simulink model "Luenberger"  (R2016a)
settings: Solver=FixedStepAuto  StartTime=0.0  StopTime=2  FixedStep=ts/20  RelTol=1e-3
values from neighbouring files (symbols this model uses):
  B = [B11 0; 0 B22; 0 0; 0 0]    [Luenberger_Parameters.m]
  B_m = [B11_m 0; 0 B22_m; 0 0; 0 0]    [Luenberger_Parameters.m]
  F = 0    [Luenberger_Parameters.m]
  J = 0.047    [Luenberger_Parameters.m]
  Lm = 0.1290    (= 0.129)    [Luenberger_Parameters.m]
  Lm_m = -err_per*Lm+Lm    (= 0.12642)    [Luenberger_Parameters.m]
  Lr = 0.1370    (= 0.137)    [Luenberger_Parameters.m]
  Lr_m = -err_per*Lr+Lr    (= 0.13426)    [Luenberger_Parameters.m]
  Ls = 0.1370    (= 0.137)    [Luenberger_Parameters.m]
  Ls_m = -err_per*Ls+Ls    (= 0.13426)    [Luenberger_Parameters.m]
  n_sync = 1500    [Luenberger_Parameters.m]
  p = 2    [Luenberger_Parameters.m]
  Rr = 1.8300    (= 1.83)    [Luenberger_Parameters.m]
  Rr_m = err_per*Rr+Rr    (= 1.8666)    [Luenberger_Parameters.m]
  Rs = 2.1900    (= 2.19)    [Luenberger_Parameters.m]
  Rs_m = err_per*Rs+Rs    (= 2.2338)    [Luenberger_Parameters.m]
  T_lim = 19    [Luenberger_Parameters.m]
  Tr_m = Lr_m/Rr_m    (= 0.0719275688417)    [Luenberger_Parameters.m]
  ts = 1/fs    (= 6.66666666667e-05)    [Luenberger_Parameters.m]
  Udc = 310    [Luenberger_Parameters.m]
undefined symbols (not defined in the file or in its folder): n_rated
settings Model: SimulationMode=accelerator  Creator=Administrator  LastModifiedBy=DELL
settings DataIOCC: LimitDataPoints=on  SaveFormat=Array  SignalLoggingSaveFormat=ModelDataLogs
settings OptimizationCC: ExpressionDepthLimit=2147483647
settings DebuggingCC: UnderspecifiedInitializationDetection=Classic  MergeDetectMultiDrivingBlocksExec=none  SolverPrmCheckMsg=warning  FcnCallInpInsideContextMsg=UseLocalSettings  StateNameClashWarn=warning
settings HardwareCC: ProdBitPerPointer=32  ProdLargestAtomicFloat=None  ProdIntDivRoundTo=Undefined  ProdEndianess=Unspecified  ProdWordSize=32  ProdHWDeviceType=32-bit Generic
settings ModelReferenceCC: PropagateSignalLabelsOutOfModel=off
settings GRTTargetCC: CombineOutputUpdateFcns=off  GRTInterface=on
settings ConfigComp: CovModelRefEnable=Off  CovSFcnEnable=off

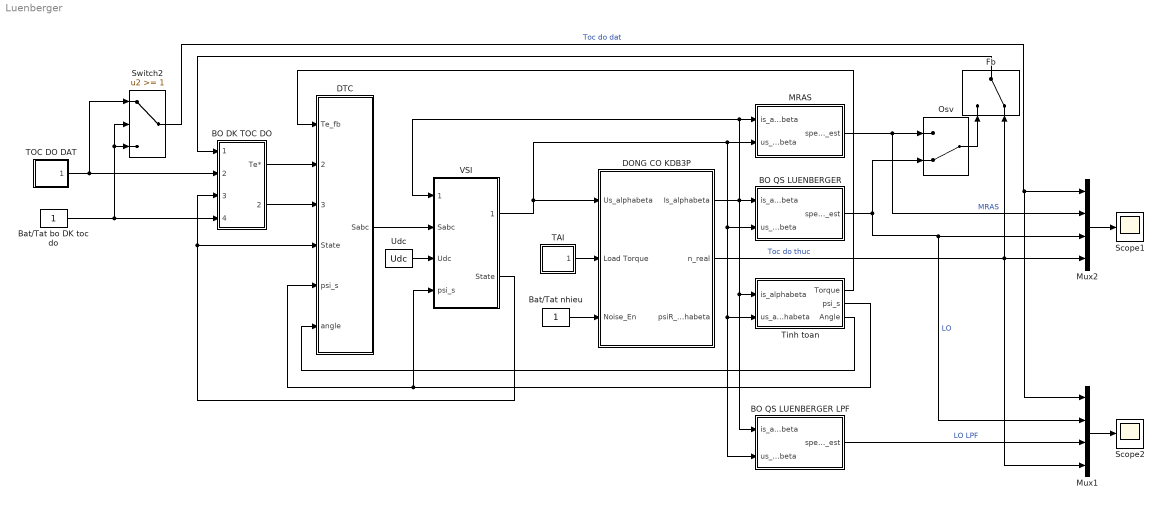
== system Luenberger ==
  BO DK TOC DO : Subsystem
  BO QS LUENBERGER : Subsystem
  BO QS LUENBERGER LPF : Subsystem
  Bat/Tat bo DK toc do : Constant
  Bat/Tat nhieu : Constant
  DONG CO KDB3P : Subsystem
  DTC : Subsystem
  Fb : ManualSwitch  CurrentSetting=0
  MRAS : Subsystem
  Mux1 : Mux
  Mux2 : Mux
  Osv : ManualSwitch  CurrentSetting=0
  Scope1 : Scope
  Scope2 : Scope
  Switch2 : Switch  Threshold=1
  TAI : Subsystem
  TOC DO DAT : Subsystem
  Tinh toan : Subsystem
  Udc : Constant  Value=Udc
  VSI : Subsystem
  wires:
  BO DK TOC DO/1(Te*) -> DTC/2(Te_ref)
  BO DK TOC DO/2(Flux*) -> DTC/3(Flux_ref)
  Tinh toan/1(Torque) -> DTC/1(Te_fb)
  Tinh toan/2(psi_s) -> DTC/5(psi_s), VSI/4(psi_s)
  VSI/2(State) -> DTC/4(State), BO DK TOC DO/3(State)
  Mux2/1 -> Scope1/1
  DTC/1(Sabc) -> VSI/2(Sabc)
  Udc/1 -> VSI/3(Udc)
  VSI/1(Us_alphabeta) -> MRAS/2(us_alphabeta), Tinh toan/2(us_alphabeta), BO QS LUENBERGER LPF/2(us_alphabeta), BO QS LUENBERGER/2(us_alphabeta), DONG CO KDB3P/1(Us_alphabeta)
  DONG CO KDB3P/1(Is_alphabeta) -> MRAS/1(is_alphabeta), VSI/1(is_alphabeta), BO QS LUENBERGER/1(is_alphabeta), BO QS LUENBERGER LPF/1(is_alphabeta), Tinh toan/1(is_alphabeta)
  Tinh toan/3(Angle) -> DTC/6(angle)
  Bat/Tat nhieu/1 -> DONG CO KDB3P/3(Noise_En)
  Fb/1 -> BO DK TOC DO/1(rpm_fb)
  Bat/Tat bo DK toc do/1 -> Switch2/3, Switch2/2, BO DK TOC DO/4(Enable)
  TOC DO DAT/1(Speed) -> Switch2/1, BO DK TOC DO/2(rpm_ref)
  TAI/1(Load) -> DONG CO KDB3P/2(Load Torque)
  MRAS/1(speed_est) -> Mux2/2, Osv/1  "MRAS"
  Osv/1 -> Fb/1
  Switch2/1 -> Mux1/1, Mux2/1  "Toc do dat"
  Mux1/1 -> Scope2/1
  DONG CO KDB3P/2(n_real) -> Mux1/4, Fb/2, Mux2/4  "Toc do thuc"
  BO QS LUENBERGER LPF/1(speed_est) -> Mux1/3  "LO LPF"
  BO QS LUENBERGER/1(speed_est) -> Mux1/2, Mux2/3, Osv/2  "LO"

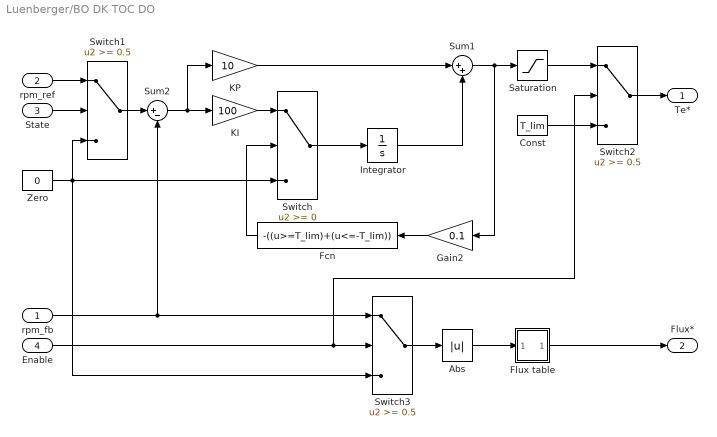
== system Luenberger/BO DK TOC DO ==
  rpm_fb : Inport
  rpm_ref : Inport  Port=2
  State : Inport  Port=3
  Enable : Inport  Port=4
  Abs : Abs  SaturateOnIntegerOverflow=on
  Const : Constant  Value=T_lim
  Fcn : Fcn  Expr=-((u>=T_lim)+(u<=-T_lim))
  Flux table : Subsystem
      mask Display: plot([0;1800;2000;2500;3000;3500], [1;1;0.90*1;0.72*1;0.6*1;0.51*1])
  Gain2 : Gain  Gain=0.1
  Integrator : Integrator  UpperSaturationLimit=T_lim  LowerSaturationLimit=-T_lim
  KI : Gain  Gain=100
  KP : Gain  Gain=10
  Saturation : Saturate  UpperLimit=T_lim  LowerLimit=-T_lim
  Sum1 : Sum  Inputs=|++
  Sum2 : Sum  Inputs=|+-
  Switch : Switch
  Switch1 : Switch  Threshold=0.5
  Switch2 : Switch  Threshold=0.5
  Switch3 : Switch  Threshold=0.5
  Zero : Constant  Value=0
  Te* : Outport
  Flux* : Outport  Port=2
  wires:
  Abs/1 -> Flux table/1(|N|)
  State/1 -> Switch1/2
  rpm_ref/1 -> Switch1/1
  Zero/1 -> Switch3/3, Switch/3, Switch1/3
  rpm_fb/1 -> Switch3/1, Sum2/2
  Switch1/1 -> Sum2/1
  Sum1/1 -> Gain2/1, Saturation/1
  KP/1 -> Sum1/1
  Fcn/1 -> Switch/2
  Gain2/1 -> Fcn/1
  Sum2/1 -> KI/1, KP/1
  Switch/1 -> Integrator/1
  KI/1 -> Switch/1
  Integrator/1 -> Sum1/2
  Saturation/1 -> Switch2/1
  Switch2/1 -> Te*/1
  Const/1 -> Switch2/3
  Flux table/1(Flux) -> Flux*/1
  Switch3/1 -> Abs/1
  Enable/1 -> Switch2/2, Switch3/2

== system Luenberger/BO QS LUENBERGER ==
  is_alphabeta : Inport
  us_alphabeta : Inport  Port=2
  Demux1 : Demux  Outputs=2
  Divide : Product  Inputs=*/
  Luenberger Adaptation Algorithm : Subsystem
  Luenberger Algorithm : Subsystem
  pole pair : Constant  Value=p
  w-->n3 : Gain  Gain=30/pi
  speed_est : Outport
  wires:
  us_alphabeta/1 -> Luenberger Algorithm/2(Us_alphabeta)
  Luenberger Adaptation Algorithm/1(wr^) -> Luenberger Algorithm/1(w_est), Divide/1
  w-->n3/1 -> speed_est/1
  Divide/1 -> w-->n3/1
  pole pair/1 -> Divide/2
  Luenberger Algorithm/1(Is_alphabeta^) -> Luenberger Adaptation Algorithm/1(is_alphabeta^)
  Luenberger Algorithm/2(PsiR_alphabeta^) -> Luenberger Adaptation Algorithm/2(psir_alphabeta^)
  is_alphabeta/1 -> Demux1/1
  Demux1/1 -> Luenberger Adaptation Algorithm/3(is_alpha), Luenberger Algorithm/3(is_alpha)
  Demux1/2 -> Luenberger Algorithm/4(is_beta), Luenberger Adaptation Algorithm/4(is_beta)

== system Luenberger/BO QS LUENBERGER LPF ==
  is_alphabeta : Inport
  us_alphabeta : Inport  Port=2
  Demux1 : Demux  Outputs=2
  Divide : Product  Inputs=*/
  Luenberger Adaptation Algorithm : Subsystem
  Luenberger Algorithm : Subsystem
  pole pair : Constant  Value=p
  w-->n3 : Gain  Gain=30/pi
  speed_est : Outport
  wires:
  us_alphabeta/1 -> Luenberger Algorithm/2(Us_alphabeta)
  Luenberger Adaptation Algorithm/1(wr^) -> Luenberger Algorithm/1(w_est), Divide/1
  w-->n3/1 -> speed_est/1
  Divide/1 -> w-->n3/1
  pole pair/1 -> Divide/2
  Luenberger Algorithm/1(Is_alphabeta^) -> Luenberger Adaptation Algorithm/1(is_alphabeta^)
  Luenberger Algorithm/2(PsiR_alphabeta^) -> Luenberger Adaptation Algorithm/2(psir_alphabeta^)
  is_alphabeta/1 -> Demux1/1
  Demux1/1 -> Luenberger Adaptation Algorithm/3(is_alpha), Luenberger Algorithm/3(is_alpha)
  Demux1/2 -> Luenberger Algorithm/4(is_beta), Luenberger Adaptation Algorithm/4(is_beta)

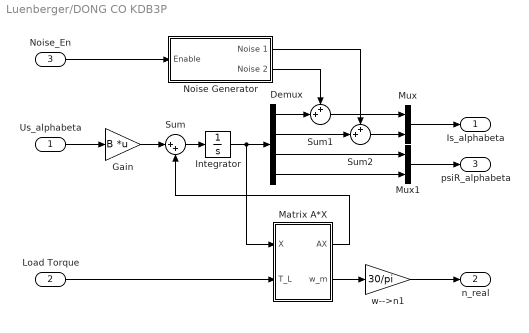
== system Luenberger/DONG CO KDB3P ==
  Us_alphabeta : Inport
  Load Torque : Inport  Port=2
  Noise_En : Inport  Port=3
  Demux : Demux
  Gain : Gain  Gain=B  Multiplication=Matrix(K*u)
  Integrator : Integrator
  Matrix A*X : Subsystem
  Mux : Mux  Inputs=2
  Mux1 : Mux  Inputs=2
  Noise Generator : Subsystem
  Sum : Sum  Inputs=|++
  Sum1 : Sum  Inputs=++|
  Sum2 : Sum  Inputs=++|
  w-->n1 : Gain  Gain=30/pi
  Is_alphabeta : Outport
  n_real : Outport  Port=2
  psiR_alphabeta : Outport  Port=3
  wires:
  Demux/3 -> Mux1/1
  Demux/4 -> Mux1/2
  Integrator/1 -> Matrix A*X/1(X), Demux/1
  Matrix A*X/1(AX) -> Sum/2
  Sum/1 -> Integrator/1
  Matrix A*X/2(w_m) -> w-->n1/1
  Us_alphabeta/1 -> Gain/1
  Gain/1 -> Sum/1
  w-->n1/1 -> n_real/1
  Load Torque/1 -> Matrix A*X/2(T_L)
  Mux1/1 -> psiR_alphabeta/1
  Mux/1 -> Is_alphabeta/1
  Demux/1 -> Sum1/2
  Demux/2 -> Sum2/2
  Sum2/1 -> Mux/2
  Sum1/1 -> Mux/1
  Noise Generator/2(Noise 2) -> Sum1/1
  Noise Generator/1(Noise 1) -> Sum2/1
  Noise_En/1 -> Noise Generator/1(Enable)

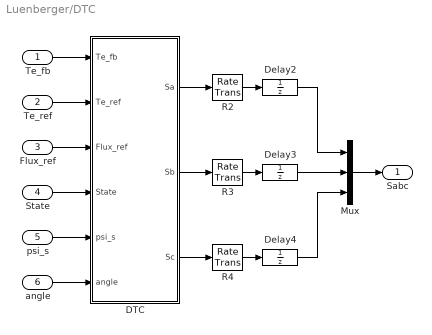
== system Luenberger/DTC ==
  Te_fb : Inport
  Te_ref : Inport  Port=2
  Flux_ref : Inport  Port=3
  State : Inport  Port=4
  psi_s : Inport  Port=5
  angle : Inport  Port=6
  DTC : MATLAB Function  TreatAsAtomicUnit=on
  Delay2 : UnitDelay  SampleTime=ts
  Delay3 : UnitDelay  SampleTime=ts
  Delay4 : UnitDelay  SampleTime=ts
  Mux : Mux  Inputs=3
  R2 : RateTransition
  R3 : RateTransition
  R4 : RateTransition
  Sabc : Outport
  wires:
  Mux/1 -> Sabc/1
  Te_fb/1 -> DTC/1(Te_fb)
  Te_ref/1 -> DTC/2(Te_ref)
  Flux_ref/1 -> DTC/3(Flux_ref)
  State/1 -> DTC/4(State)
  psi_s/1 -> DTC/5(psi_s)
  angle/1 -> DTC/6(angle)
  DTC/1(Sa) -> R2/1
  DTC/2(Sb) -> R3/1
  DTC/3(Sc) -> R4/1
  R2/1 -> Delay2/1
  R3/1 -> Delay3/1
  R4/1 -> Delay4/1
  Delay2/1 -> Mux/1
  Delay3/1 -> Mux/2
  Delay4/1 -> Mux/3

== system Luenberger/MRAS ==
  is_alphabeta : Inport
  us_alphabeta : Inport  Port=2
  CB Adaptation Algorithm : Subsystem
  CB Adaptive Model : Subsystem
  CB Estimator : Subsystem
  Divide : Product  Inputs=*/
  Lm measured : Constant  Value=Lm_m
  Lr measured : Constant  Value=Lr_m
  Ls measured : Constant  Value=Ls_m
  Rr measured : Constant  Value=Rr_m
  Rs measured : Constant  Value=Rs_m
  pole pair : Constant  Value=p
  w-->n3 : Gain  Gain=30/pi
  speed_est : Outport
  wires:
  us_alphabeta/1 -> CB Estimator/1(us_alphabeta)
  CB Adaptation Algorithm/1(w_r_CB^) -> Divide/1, CB Estimator/2(w_r_CB^), CB Adaptive Model/2(w_r_CB^)
  CB Estimator/1(is_alphabeta^) -> CB Adaptation Algorithm/1(is_alphabeta^)
  CB Adaptive Model/1(psir_alpha^) -> CB Adaptation Algorithm/3(psir_alpha^), CB Estimator/8(psir_alpha^)
  is_alphabeta/1 -> CB Adaptive Model/1(is_alphabeta), CB Adaptation Algorithm/2(is_alphabeta)
  Lm measured/1 -> CB Estimator/3("Lm_m ")
  Lr measured/1 -> CB Estimator/4(Lr_m)
  Ls measured/1 -> CB Estimator/5(Ls_m)
  Rr measured/1 -> CB Estimator/6(Rr_m)
  Rs measured/1 -> CB Estimator/7(Rs_m)
  CB Adaptive Model/2(psir_beta^) -> CB Adaptation Algorithm/4(psir_beta^), CB Estimator/9(psir_beta^)
  w-->n3/1 -> speed_est/1
  Divide/1 -> w-->n3/1
  pole pair/1 -> Divide/2

== system Luenberger/TAI ==
  note: Select=0: No load
      | Select=1: 10% load
      | Select=2: 0% -100% load
      | Select>2: 0%, 10%, 50%, 80% load
  Clock : Clock
  Load Generator : MATLAB Function  TreatAsAtomicUnit=on
  Select : Constant  Value=2
  Tmax : Constant  Value=T_lim
  Load : Outport
  wires:
  Load Generator/1(T_Load) -> Load/1
  Select/1 -> Load Generator/1(Select)
  Tmax/1 -> Load Generator/2(Tmax)
  Clock/1 -> Load Generator/3(t)

== system Luenberger/TOC DO DAT ==
  note: Select=1: 100rpm
      | Select=2: 500rpm
      | Select>2: 1000, 500, 100rpm
  Clock : Clock
  Select : Constant  Value=3
  Speed Selection : MATLAB Function  TreatAsAtomicUnit=on
  Speed : Outport
  wires:
  Speed Selection/1(Speed) -> Speed/1
  Select/1 -> Speed Selection/1(Select)
  Clock/1 -> Speed Selection/2(t)

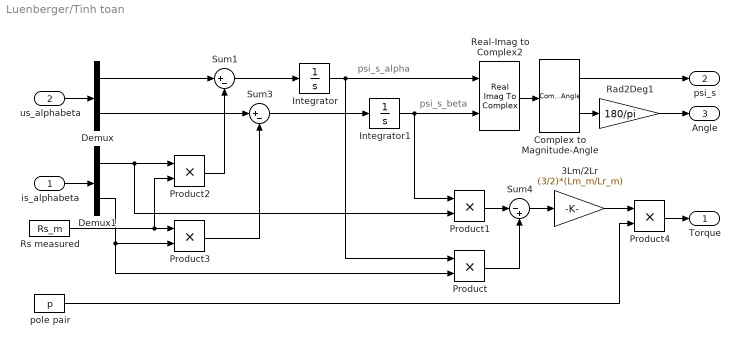
== system Luenberger/Tinh toan ==
  note: psi_s_beta
  note: psi_s_alpha
  is_alphabeta : Inport
  us_alphabeta : Inport  Port=2
  3Lm/2Lr : Gain  Gain=(3/2)*(Lm_m/Lr_m)
  Complex to Magnitude-Angle : ComplexToMagnitudeAngle
  Demux : Demux  Outputs=2
  Demux1 : Demux  Outputs=2
  Integrator : Integrator
  Integrator1 : Integrator  LimitOutput=on  UpperSaturationLimit=pi  LowerSaturationLimit=-pi
  Product{,1..4} (5 alike) : Product  RndMeth=Zero
  Rad2Deg1 : Gain  Gain=180/pi
  Real-Imag to Complex2 : RealImagToComplex
  Rs measured : Constant  Value=Rs_m
  Sum1 : Sum  Inputs=|+-
  Sum3 : Sum  Inputs=|+-
  Sum4 : Sum  Inputs=|-+
  pole pair : Constant  Value=p
  Torque : Outport
  psi_s : Outport  Port=2
  Angle : Outport  Port=3
  wires:
  Product2/1 -> Sum1/2
  Sum1/1 -> Integrator/1
  Integrator/1 -> Real-Imag to Complex2/1, Product/1
  Product3/1 -> Sum3/2
  Sum3/1 -> Integrator1/1
  Demux/2 -> Sum3/1
  Demux1/2 -> Product/2, Product3/2
  Product1/1 -> Sum4/1
  Product/1 -> Sum4/2
  Sum4/1 -> 3Lm/2Lr/1
  Real-Imag to Complex2/1 -> Complex to Magnitude-Angle/1
  Complex to Magnitude-Angle/1 -> psi_s/1
  Rs measured/1 -> Product2/2, Product3/1
  Demux/1 -> Sum1/1
  us_alphabeta/1 -> Demux/1
  is_alphabeta/1 -> Demux1/1
  Demux1/1 -> Product1/2, Product2/1
  Integrator1/1 -> Product1/1, Real-Imag to Complex2/2
  pole pair/1 -> Product4/2
  3Lm/2Lr/1 -> Product4/1
  Product4/1 -> Torque/1
  Rad2Deg1/1 -> Angle/1
  Complex to Magnitude-Angle/2 -> Rad2Deg1/1

== system Luenberger/VSI ==
  is_alphabeta : Inport
  Sabc : Inport  Port=2
  Udc : Inport  Port=3
  psi_s : Inport  Port=4
  Delay : UnitDelay  SampleTime=ts
  Demux : Demux  Outputs=3
  Demux1 : Demux  Outputs=2
  Mux : Mux  Inputs=2
  R5 : RateTransition
  VSI : MATLAB Function  TreatAsAtomicUnit=on
  Us_alphabeta : Outport
  State : Outport  Port=2
  wires:
  Udc/1 -> VSI/4(Udc)
  VSI/3(State) -> State/1, R5/1
  Delay/1 -> VSI/8(Start)
  R5/1 -> Delay/1
  Sabc/1 -> Demux/1
  Demux/1 -> VSI/1(Sa)
  Demux/2 -> VSI/2(Sb)
  psi_s/1 -> VSI/5(psi_s)
  Mux/1 -> Us_alphabeta/1
  VSI/1(u_alpha) -> Mux/1
  VSI/2(u_beta) -> Mux/2
  Demux/3 -> VSI/3(Sc)
  is_alphabeta/1 -> Demux1/1
  Demux1/1 -> VSI/6(is_alpha)
  Demux1/2 -> VSI/7(is_beta)

== system Luenberger/BO DK TOC DO/Flux table ==
  |N| : Inport
  Abs1 : Abs  SaturateOnIntegerOverflow=on
  F : Fcn  Expr=n_sync*0.78/u(1)
  Saturation : Saturate  UpperLimit=inf  LowerLimit=1500
  Flux : Outport
  wires:
  Abs1/1 -> Saturation/1
  F/1 -> Flux/1
  |N|/1 -> Abs1/1
  Saturation/1 -> F/1

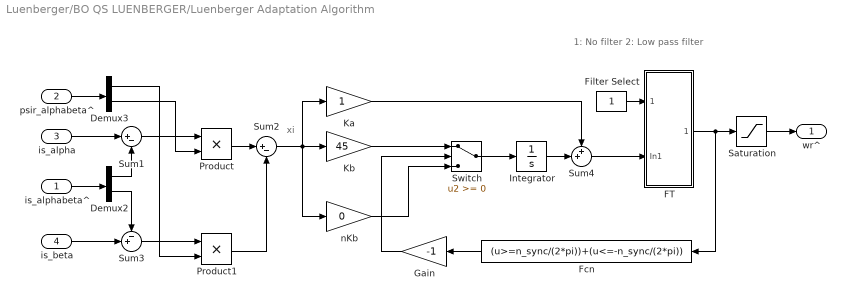
== system Luenberger/BO QS LUENBERGER/Luenberger Adaptation Algorithm ==
  note: 1: No filter
      | 2: Low pass filter
  note: xi
  is_alphabeta^ : Inport
  psir_alphabeta^ : Inport  Port=2
  is_alpha : Inport  Port=3
  is_beta : Inport  Port=4
  Demux2 : Demux  Outputs=2
  Demux3 : Demux  Outputs=2
  FT : Subsystem
  Fcn : Fcn  Expr=(u>=n_sync/(2*pi))+(u<=-n_sync/(2*pi))
  Filter Select : Constant
  Gain : Gain  Gain=-1
  Integrator : Integrator  UpperSaturationLimit=n_rated/(2*pi)  LowerSaturationLimit=-n_rated/(2*pi)
  Ka : Gain
  Kb : Gain  Gain=45
  Product : Product  RndMeth=Zero
  Product1 : Product  RndMeth=Zero
  Saturation : Saturate  UpperLimit=n_sync/(2*pi)  LowerLimit=-n_sync/(2*pi)
  Sum1 : Sum  Inputs=|+-
  Sum2 : Sum  Inputs=|+-
  Sum3 : Sum  Inputs=-+|
  Sum4 : Sum  Inputs=++|
  Switch : Switch
  nKb : Gain  Gain=0
  wr^ : Outport
  wires:
  Product1/1 -> Sum2/2
  Demux3/2 -> Product/2
  Demux3/1 -> Product1/2
  Product/1 -> Sum2/1
  Integrator/1 -> Sum4/2
  Switch/1 -> Integrator/1
  is_alphabeta^/1 -> Demux2/1
  psir_alphabeta^/1 -> Demux3/1
  Sum1/1 -> Product/1
  Sum3/1 -> Product1/1
  Filter Select/1 -> FT/1(Select)
  Demux2/2 -> Sum3/1
  is_beta/1 -> Sum3/2
  Demux2/1 -> Sum1/2
  is_alpha/1 -> Sum1/1
  Sum2/1 -> Ka/1, nKb/1, Kb/1
  Kb/1 -> Switch/1
  Fcn/1 -> Gain/1
  Gain/1 -> Switch/2
  nKb/1 -> Switch/3
  Saturation/1 -> wr^/1
  Ka/1 -> Sum4/1
  Sum4/1 -> FT/2(In1)
  FT/1(Out1) -> Fcn/1, Saturation/1

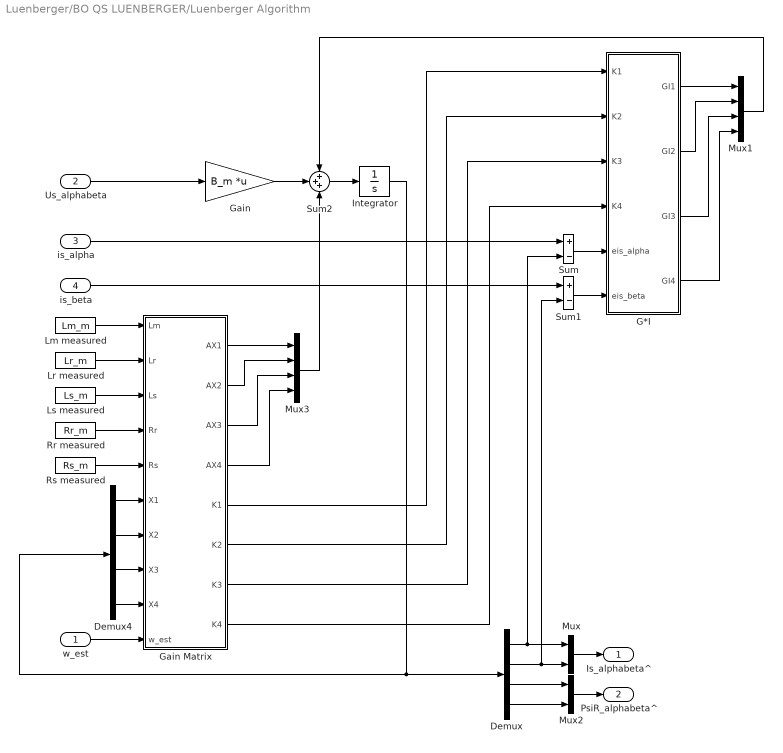
== system Luenberger/BO QS LUENBERGER/Luenberger Algorithm ==
  w_est : Inport
  Us_alphabeta : Inport  Port=2
  is_alpha : Inport  Port=3
  is_beta : Inport  Port=4
  Demux : Demux
  Demux4 : Demux
  G*I : MATLAB Function  TreatAsAtomicUnit=on
  Gain : Gain  Gain=B_m  Multiplication=Matrix(K*u)
  Gain Matrix : MATLAB Function  TreatAsAtomicUnit=on
  Integrator : Integrator
  Lm measured : Constant  Value=Lm_m
  Lr measured : Constant  Value=Lr_m
  Ls measured : Constant  Value=Ls_m
  Mux : Mux  Inputs=2
  Mux1 : Mux
  Mux2 : Mux  Inputs=2
  Mux3 : Mux
  Rr measured : Constant  Value=Rr_m
  Rs measured : Constant  Value=Rs_m
  Sum : Sum  Inputs=+-
  Sum1 : Sum  Inputs=+-
  Sum2 : Sum  Inputs=+++
  Is_alphabeta^ : Outport
  PsiR_alphabeta^ : Outport  Port=2
  wires:
  Demux/1 -> Mux/1, Sum/2
  Demux/2 -> Mux/2, Sum1/2
  Sum2/1 -> Integrator/1
  Mux1/1 -> Sum2/1
  Sum/1 -> G*I/5(eis_alpha)
  Sum1/1 -> G*I/6(eis_beta)
  G*I/1(GI1) -> Mux1/1
  G*I/2(GI2) -> Mux1/2
  G*I/3(GI3) -> Mux1/3
  G*I/4(GI4) -> Mux1/4
  is_alpha/1 -> Sum/1
  is_beta/1 -> Sum1/1
  Mux/1 -> Is_alphabeta^/1
  Demux/3 -> Mux2/1
  Demux/4 -> Mux2/2
  Mux2/1 -> PsiR_alphabeta^/1
  Gain/1 -> Sum2/2
  Us_alphabeta/1 -> Gain/1
  Integrator/1 -> Demux4/1, Demux/1
  Demux4/2 -> Gain Matrix/7(X2)
  Demux4/3 -> Gain Matrix/8(X3)
  Demux4/1 -> Gain Matrix/6(X1)
  Demux4/4 -> Gain Matrix/9(X4)
  Gain Matrix/1(AX1) -> Mux3/1
  Gain Matrix/2(AX2) -> Mux3/2
  Gain Matrix/3(AX3) -> Mux3/3
  Gain Matrix/4(AX4) -> Mux3/4
  Gain Matrix/8(K4) -> G*I/4(K4)
  Gain Matrix/7(K3) -> G*I/3(K3)
  Gain Matrix/6(K2) -> G*I/2(K2)
  Gain Matrix/5(K1) -> G*I/1(K1)
  Mux3/1 -> Sum2/3
  Lm measured/1 -> Gain Matrix/1(Lm)
  Lr measured/1 -> Gain Matrix/2(Lr)
  Ls measured/1 -> Gain Matrix/3(Ls)
  Rr measured/1 -> Gain Matrix/4(Rr)
  Rs measured/1 -> Gain Matrix/5(Rs)
  w_est/1 -> Gain Matrix/10(w_est)

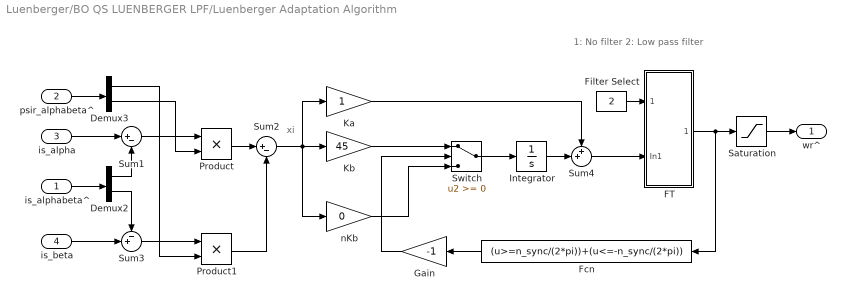
== system Luenberger/BO QS LUENBERGER LPF/Luenberger Adaptation Algorithm ==
  note: 1: No filter
      | 2: Low pass filter
  note: xi
  is_alphabeta^ : Inport
  psir_alphabeta^ : Inport  Port=2
  is_alpha : Inport  Port=3
  is_beta : Inport  Port=4
  Demux2 : Demux  Outputs=2
  Demux3 : Demux  Outputs=2
  FT : Subsystem
  Fcn : Fcn  Expr=(u>=n_sync/(2*pi))+(u<=-n_sync/(2*pi))
  Filter Select : Constant  Value=2
  Gain : Gain  Gain=-1
  Integrator : Integrator  UpperSaturationLimit=n_rated/(2*pi)  LowerSaturationLimit=-n_rated/(2*pi)
  Ka : Gain
  Kb : Gain  Gain=45
  Product : Product  RndMeth=Zero
  Product1 : Product  RndMeth=Zero
  Saturation : Saturate  UpperLimit=n_sync/(2*pi)  LowerLimit=-n_sync/(2*pi)
  Sum1 : Sum  Inputs=|+-
  Sum2 : Sum  Inputs=|+-
  Sum3 : Sum  Inputs=-+|
  Sum4 : Sum  Inputs=++|
  Switch : Switch
  nKb : Gain  Gain=0
  wr^ : Outport
  wires:
  Product1/1 -> Sum2/2
  Demux3/2 -> Product/2
  Demux3/1 -> Product1/2
  Product/1 -> Sum2/1
  Integrator/1 -> Sum4/2
  Switch/1 -> Integrator/1
  is_alphabeta^/1 -> Demux2/1
  psir_alphabeta^/1 -> Demux3/1
  Sum1/1 -> Product/1
  Sum3/1 -> Product1/1
  Filter Select/1 -> FT/1(Select)
  Demux2/2 -> Sum3/1
  is_beta/1 -> Sum3/2
  Demux2/1 -> Sum1/2
  is_alpha/1 -> Sum1/1
  Sum2/1 -> Ka/1, nKb/1, Kb/1
  Kb/1 -> Switch/1
  Fcn/1 -> Gain/1
  Gain/1 -> Switch/2
  nKb/1 -> Switch/3
  Saturation/1 -> wr^/1
  Ka/1 -> Sum4/1
  Sum4/1 -> FT/2(In1)
  FT/1(Out1) -> Fcn/1, Saturation/1

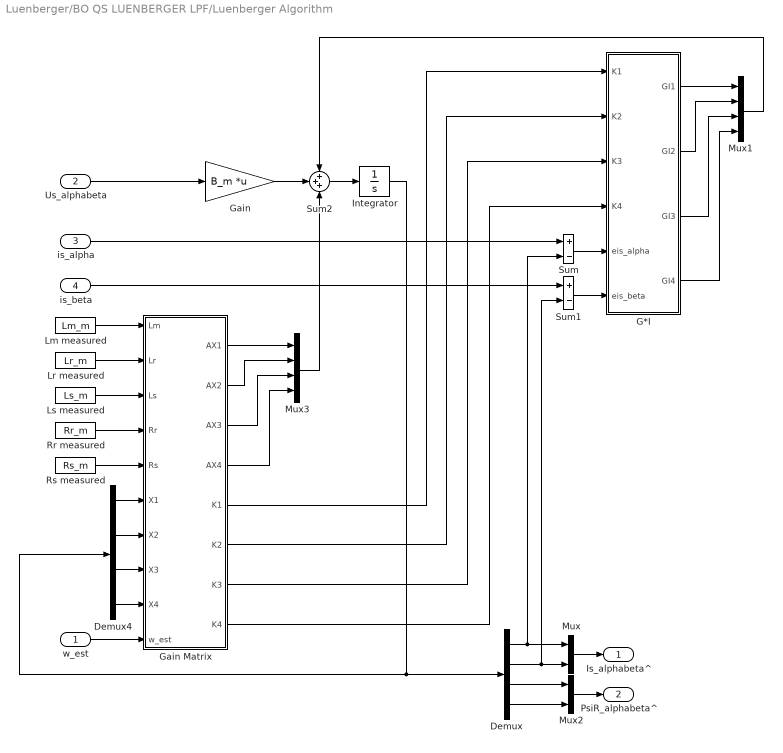
== system Luenberger/BO QS LUENBERGER LPF/Luenberger Algorithm ==
  w_est : Inport
  Us_alphabeta : Inport  Port=2
  is_alpha : Inport  Port=3
  is_beta : Inport  Port=4
  Demux : Demux
  Demux4 : Demux
  G*I : MATLAB Function  TreatAsAtomicUnit=on
  Gain : Gain  Gain=B_m  Multiplication=Matrix(K*u)
  Gain Matrix : MATLAB Function  TreatAsAtomicUnit=on
  Integrator : Integrator
  Lm measured : Constant  Value=Lm_m
  Lr measured : Constant  Value=Lr_m
  Ls measured : Constant  Value=Ls_m
  Mux : Mux  Inputs=2
  Mux1 : Mux
  Mux2 : Mux  Inputs=2
  Mux3 : Mux
  Rr measured : Constant  Value=Rr_m
  Rs measured : Constant  Value=Rs_m
  Sum : Sum  Inputs=+-
  Sum1 : Sum  Inputs=+-
  Sum2 : Sum  Inputs=+++
  Is_alphabeta^ : Outport
  PsiR_alphabeta^ : Outport  Port=2
  wires:
  Demux/1 -> Mux/1, Sum/2
  Demux/2 -> Mux/2, Sum1/2
  Sum2/1 -> Integrator/1
  Mux1/1 -> Sum2/1
  Sum/1 -> G*I/5(eis_alpha)
  Sum1/1 -> G*I/6(eis_beta)
  G*I/1(GI1) -> Mux1/1
  G*I/2(GI2) -> Mux1/2
  G*I/3(GI3) -> Mux1/3
  G*I/4(GI4) -> Mux1/4
  is_alpha/1 -> Sum/1
  is_beta/1 -> Sum1/1
  Mux/1 -> Is_alphabeta^/1
  Demux/3 -> Mux2/1
  Demux/4 -> Mux2/2
  Mux2/1 -> PsiR_alphabeta^/1
  Gain/1 -> Sum2/2
  Us_alphabeta/1 -> Gain/1
  Integrator/1 -> Demux4/1, Demux/1
  Demux4/2 -> Gain Matrix/7(X2)
  Demux4/3 -> Gain Matrix/8(X3)
  Demux4/1 -> Gain Matrix/6(X1)
  Demux4/4 -> Gain Matrix/9(X4)
  Gain Matrix/1(AX1) -> Mux3/1
  Gain Matrix/2(AX2) -> Mux3/2
  Gain Matrix/3(AX3) -> Mux3/3
  Gain Matrix/4(AX4) -> Mux3/4
  Gain Matrix/8(K4) -> G*I/4(K4)
  Gain Matrix/7(K3) -> G*I/3(K3)
  Gain Matrix/6(K2) -> G*I/2(K2)
  Gain Matrix/5(K1) -> G*I/1(K1)
  Mux3/1 -> Sum2/3
  Lm measured/1 -> Gain Matrix/1(Lm)
  Lr measured/1 -> Gain Matrix/2(Lr)
  Ls measured/1 -> Gain Matrix/3(Ls)
  Rr measured/1 -> Gain Matrix/4(Rr)
  Rs measured/1 -> Gain Matrix/5(Rs)
  w_est/1 -> Gain Matrix/10(w_est)

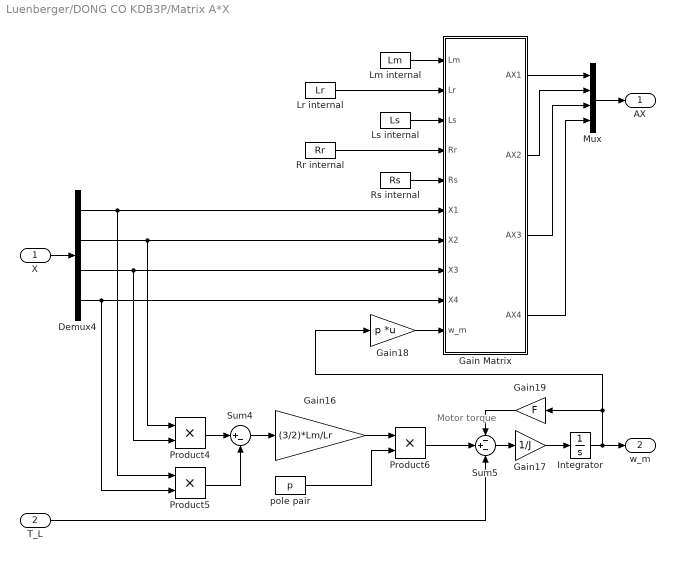
== system Luenberger/DONG CO KDB3P/Matrix A*X ==
  note: Motor
      | torque
  X : Inport
  T_L : Inport  Port=2
  Demux4 : Demux
  Gain Matrix : MATLAB Function  TreatAsAtomicUnit=on
  Gain16 : Gain  Gain=(3/2)*Lm/Lr
  Gain17 : Gain  Gain=1/J
  Gain18 : Gain  Gain=p  Multiplication=Matrix(K*u)
  Gain19 : Gain  Gain=F
  Integrator : Integrator
  Lm internal : Constant  Value=Lm
  Lr internal : Constant  Value=Lr
  Ls internal : Constant  Value=Ls
  Mux : Mux
  Product4 : Product  RndMeth=Zero
  Product5 : Product  RndMeth=Zero
  Product6 : Product  RndMeth=Zero
  Rr internal : Constant  Value=Rr
  Rs internal : Constant  Value=Rs
  Sum4 : Sum  Inputs=|+-
  Sum5 : Sum  Inputs=-+-
  pole pair : Constant  Value=p
  AX : Outport
  w_m : Outport  Port=2
  wires:
  X/1 -> Demux4/1
  Mux/1 -> AX/1
  Product5/1 -> Sum4/2
  Product4/1 -> Sum4/1
  Sum4/1 -> Gain16/1
  Demux4/2 -> Product4/1, Gain Matrix/7(X2)
  Demux4/3 -> Product4/2, Gain Matrix/8(X3)
  Demux4/1 -> Product5/1, Gain Matrix/6(X1)
  Demux4/4 -> Gain Matrix/9(X4), Product5/2
  Gain16/1 -> Product6/1
  pole pair/1 -> Product6/2
  Product6/1 -> Sum5/2
  Sum5/1 -> Gain17/1
  Gain17/1 -> Integrator/1
  Integrator/1 -> w_m/1, Gain18/1, Gain19/1
  T_L/1 -> Sum5/3
  Gain19/1 -> Sum5/1
  Gain Matrix/1(AX1) -> Mux/1
  Gain Matrix/2(AX2) -> Mux/2
  Gain Matrix/3(AX3) -> Mux/3
  Gain Matrix/4(AX4) -> Mux/4
  Gain18/1 -> Gain Matrix/10(w_m)
  Lm internal/1 -> Gain Matrix/1(Lm)
  Lr internal/1 -> Gain Matrix/2(Lr)
  Ls internal/1 -> Gain Matrix/3(Ls)
  Rr internal/1 -> Gain Matrix/4(Rr)
  Rs internal/1 -> Gain Matrix/5(Rs)

== system Luenberger/DONG CO KDB3P/Noise Generator ==
  Enable : Inport
  Constant : Constant  Value=0
  Gain1 : Gain  Gain=0.05
  Gain2 : Gain  Gain=0.01
  Switch : Switch  Criteria=u2 > Threshold
  Switch1 : Switch  Criteria=u2 > Threshold  Threshold=1
  White Noise : RandomNumber  DisableCoverage=on  Mean=1  Seed=[65536]  SampleTime=[0 0]
  White Noise1 : RandomNumber  DisableCoverage=on  Mean=1  Seed=[65536]  SampleTime=[0 0]
  Noise 1 : Outport
  Noise 2 : Outport  Port=2
  wires:
  White Noise/1 -> Gain1/1
  White Noise1/1 -> Gain2/1
  Gain1/1 -> Switch1/1
  Switch1/1 -> Noise 1/1
  Gain2/1 -> Switch/1
  Switch/1 -> Noise 2/1
  Enable/1 -> Switch/2, Switch1/2
  Constant/1 -> Switch1/3, Switch/3

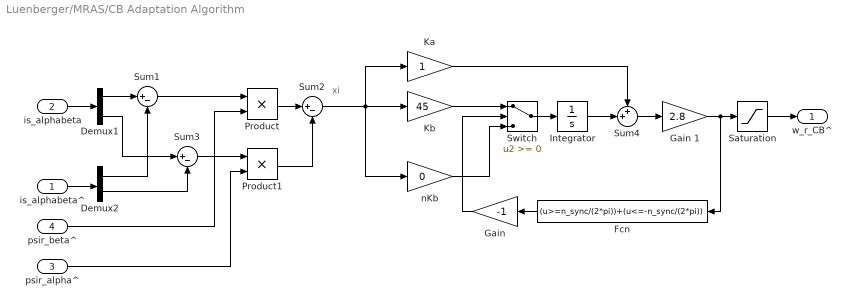
== system Luenberger/MRAS/CB Adaptation Algorithm ==
  note: xi
  is_alphabeta^ : Inport
  is_alphabeta : Inport  Port=2
  psir_alpha^ : Inport  Port=3
  psir_beta^ : Inport  Port=4
  Demux1 : Demux  Outputs=2
  Demux2 : Demux  Outputs=2
  Fcn : Fcn  Expr=(u>=n_sync/(2*pi))+(u<=-n_sync/(2*pi))
  Gain : Gain  Gain=-1
  Gain 1 : Gain  Gain=2.8
  Integrator : Integrator  UpperSaturationLimit=n_rated/(2*pi)  LowerSaturationLimit=-n_rated/(2*pi)
  Ka : Gain
  Kb : Gain  Gain=45
  Product : Product  RndMeth=Zero
  Product1 : Product  RndMeth=Zero
  Saturation : Saturate  UpperLimit=n_sync/(2*pi)  LowerLimit=-n_sync/(2*pi)
  Sum1 : Sum  Inputs=|+-
  Sum2 : Sum  Inputs=|+-
  Sum3 : Sum  Inputs=|+-
  Sum4 : Sum  Inputs=++|
  Switch : Switch
  nKb : Gain  Gain=0
  w_r_CB^ : Outport
  wires:
  Product1/1 -> Sum2/2
  Sum2/1 -> Ka/1, nKb/1, Kb/1
  Demux1/1 -> Sum1/1
  Demux2/1 -> Sum1/2
  Sum1/1 -> Product/1
  psir_beta^/1 -> Product/2
  Demux1/2 -> Sum3/1
  Demux2/2 -> Sum3/2
  Sum3/1 -> Product1/1
  psir_alpha^/1 -> Product1/2
  Product/1 -> Sum2/1
  Saturation/1 -> w_r_CB^/1
  is_alphabeta/1 -> Demux1/1
  is_alphabeta^/1 -> Demux2/1
  Integrator/1 -> Sum4/2
  Switch/1 -> Integrator/1
  Kb/1 -> Switch/1
  Fcn/1 -> Gain/1
  Gain/1 -> Switch/2
  nKb/1 -> Switch/3
  Ka/1 -> Sum4/1
  Sum4/1 -> Gain 1/1
  Gain 1/1 -> Fcn/1, Saturation/1

== system Luenberger/MRAS/CB Adaptive Model ==
  is_alphabeta : Inport
  w_r_CB^ : Inport  Port=2
  Demux : Demux  Outputs=2
  Integrator : Integrator
  Integrator1 : Integrator
  Lm_Tr : Gain  Gain=Lm_m/Tr_m
  Lm_Tr1 : Gain  Gain=Lm_m/Tr_m
  Product : Product  RndMeth=Zero
  Product1 : Product  RndMeth=Zero
  Sum1 : Sum  Inputs=+--
  Sum2 : Sum  Inputs=-++
  Tr : Gain  Gain=1/Tr_m
  Tr1 : Gain  Gain=1/Tr_m
  psir_alpha^ : Outport
  psir_beta^ : Outport  Port=2
  wires:
  Lm_Tr1/1 -> Sum2/3
  Demux/2 -> Lm_Tr1/1
  Sum2/1 -> Integrator/1
  Sum1/1 -> Integrator1/1
  w_r_CB^/1 -> Product/2, Product1/2
  Integrator/1 -> psir_beta^/1, Tr1/1, Product/1
  Integrator1/1 -> psir_alpha^/1, Tr/1, Product1/1
  Tr1/1 -> Sum2/1
  Product1/1 -> Sum2/2
  Product/1 -> Sum1/2
  Lm_Tr/1 -> Sum1/1
  Tr/1 -> Sum1/3
  Demux/1 -> Lm_Tr/1
  is_alphabeta/1 -> Demux/1

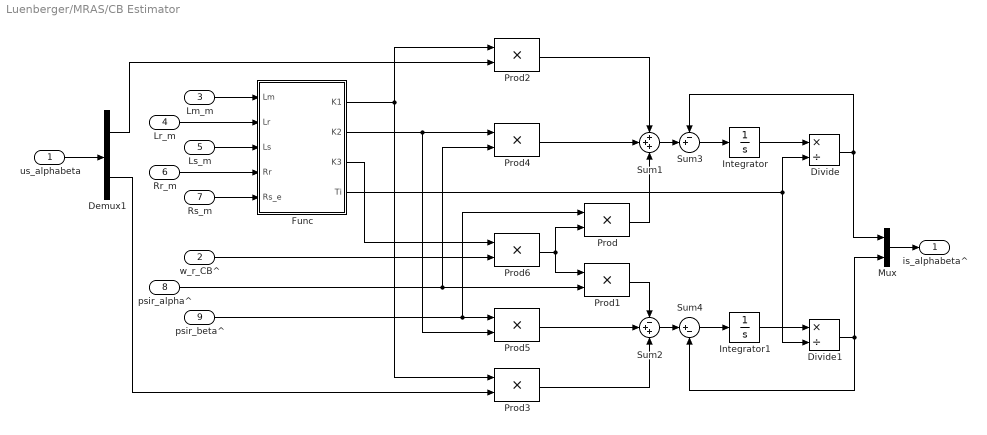
== system Luenberger/MRAS/CB Estimator ==
  us_alphabeta : Inport
  w_r_CB^ : Inport  Port=2
  "Lm_m " : Inport  Port=3
  Lr_m : Inport  Port=4
  Ls_m : Inport  Port=5
  Rr_m : Inport  Port=6
  Rs_m : Inport  Port=7
  psir_alpha^ : Inport  Port=8
  psir_beta^ : Inport  Port=9
  Demux1 : Demux  Outputs=2
  Divide : Product  Inputs=*/
  Divide1 : Product  Inputs=*/
  Func : MATLAB Function  TreatAsAtomicUnit=on
  Integrator : Integrator
  Integrator1 : Integrator
  Mux : Mux  Inputs=2
  Prod{,1..6} (7 alike) : Product  RndMeth=Zero
  Sum1 : Sum  Inputs=+++
  Sum2 : Sum  Inputs=-++
  Sum3 : Sum  Inputs=-+|
  Sum4 : Sum  Inputs=|+-
  is_alphabeta^ : Outport
  wires:
  Divide1/1 -> Mux/2, Sum4/2
  Integrator1/1 -> Divide1/1
  Sum4/1 -> Integrator1/1
  Func/4(Ti) -> Divide1/2, Divide/2
  Divide/1 -> Mux/1, Sum3/1
  Integrator/1 -> Divide/1
  Sum3/1 -> Integrator/1
  Func/3(K3) -> Prod6/1
  Func/2(K2) -> Prod5/2, Prod4/1
  Prod3/1 -> Sum2/3
  Demux1/2 -> Prod3/2
  Func/1(K1) -> Prod2/1, Prod3/1
  Rs_m/1 -> Func/5(Rs_e)
  Prod2/1 -> Sum1/1
  Prod4/1 -> Sum1/2
  Prod/1 -> Sum1/3
  Prod5/1 -> Sum2/2
  Prod1/1 -> Sum2/1
  Prod6/1 -> Prod/2, Prod1/1
  w_r_CB^/1 -> Prod6/2
  Sum2/1 -> Sum4/1
  "Lm_m "/1 -> Func/1(Lm)
  Lr_m/1 -> Func/2(Lr)
  Ls_m/1 -> Func/3(Ls)
  Rr_m/1 -> Func/4(Rr)
  Sum1/1 -> Sum3/2
  us_alphabeta/1 -> Demux1/1
  Demux1/1 -> Prod2/2
  psir_beta^/1 -> Prod/1, Prod5/1
  psir_alpha^/1 -> Prod4/2, Prod1/2
  Mux/1 -> is_alphabeta^/1

== system Luenberger/BO QS LUENBERGER/Luenberger Adaptation Algorithm/FT ==
  Select : Inport
  In1 : Inport  Port=2
  Gain : Gain  Gain=1.4
  LPF : MATLAB Function  TreatAsAtomicUnit=on
  Multiport Switch : MultiPortSwitch  Inputs=2
  Out1 : Outport
  wires:
  Select/1 -> Multiport Switch/1
  LPF/1(y) -> Multiport Switch/3
  In1/1 -> Multiport Switch/2, LPF/1(u)
  Multiport Switch/1 -> Gain/1
  Gain/1 -> Out1/1

== system Luenberger/BO QS LUENBERGER LPF/Luenberger Adaptation Algorithm/FT ==
  Select : Inport
  In1 : Inport  Port=2
  Gain : Gain  Gain=1.4
  LPF : MATLAB Function  TreatAsAtomicUnit=on
  Multiport Switch : MultiPortSwitch  Inputs=2
  Out1 : Outport
  wires:
  Select/1 -> Multiport Switch/1
  LPF/1(y) -> Multiport Switch/3
  In1/1 -> Multiport Switch/2, LPF/1(u)
  Multiport Switch/1 -> Gain/1
  Gain/1 -> Out1/1

== matlab function Luenberger/TAI/Load Generator ==
  data: Select input; T_Load output; Tmax input; t input
function T_Load = fcn(Select, Tmax, t)

switch Select
    case 0 % No load
        T_Load=0;
        
    case 1 % 10% Load
        T_Load=0.1*Tmax;
        
    case 2 % 0%->100% Load
        T_Load=0.1*Tmax*t;
        if T_Load>Tmax
            T_Load=Tmax;
        end
        
    otherwise % 0%, 10%, 50%, 80%
        if t<0.5
            T_Load=0;
        elseif t<1.0
            T_Load=0.1*Tmax;
        elseif t<1.5
            T_Load=0.5*Tmax;
        else
            T_Load=0.8*Tmax;
        end
end

== matlab function Luenberger/DONG CO KDB3P/Matrix A*X/Gain Matrix ==
  data: Lm input; Lr input; Ls input; Rr input; Rs input; X1 input; AX1 output; X2 input; X3 input; X4 input; w_m input; AX2 output; AX3 output; AX4 output
function [AX1,AX2,AX3,AX4] = fcn(Lm, Lr, Ls, Rr, Rs, X1, X2, X3, X4, w_m)

sigma=1-(Lm^2)/(Ls*Lr);

A11=-(Lm^2*Rr+Lr^2*Rs)/(sigma*Ls*Lr^2);
A12=0;
A13=Lm*Rr/(sigma*Ls*Lr^2);
A14=Lm/(sigma*Ls*Lr);
A21=0;
A22=A11;
A23=-A14;
A24=A13;
A31=Lm*Rr/Lr;
A32=0;
A33=-Rr/Lr;
A34=-1;
A41=0;
A42=A31;
A43=-A34;
A44=A33;

AX1=X1*A11+X2*A12+X3*A13+X4*w_m*A14;
AX2=X1*A21+X2*A22+X3*w_m*A23+X4*A24;
AX3=X1*A31+X2*A32+X3*A33+X4*w_m*A34;
AX4=X1*A41+X2*A42+X3*w_m*A43+X4*A44;

== matlab function Luenberger/VSI/VSI ==
  data: Sa input; Sb input; Sc input; u_alpha output; Udc input; psi_s input; is_alpha input; is_beta input; u_beta output; Start input; State output
function [u_alpha, u_beta, State] = fcn(Sa, Sb, Sc, Udc, psi_s, is_alpha, is_beta, Start)

% is_beta is unused

u_alpha=0;
u_beta=0;
u_b=0;
u_c=0;

if Start==0
    if psi_s>=-0.22
        State=1;
        
    else
        State=0;
        u_alpha=(2/3)*Udc;
            u_b=(-1/3)*Udc;
            u_c=(-1/3)*Udc;
        if is_alpha<8.0
            u_alpha=(2/3)*Udc;
            u_b=(-1/3)*Udc;
            u_c=(-1/3)*Udc;
        end;

        if is_alpha>=10.0
            u_alpha=0;
            u_b=0;
            u_c=0;
        end;
    
            
    end;
    
    u_beta=(u_alpha+2*u_b)/sqrt(3);

  
else
 
    State=1;
    if Sa==0 && Sb==0 && Sc==0
        u_alpha=0;u_b=0;u_c=0;
    elseif Sa==1 && Sb==1 && Sc==1
        u_alpha=0;u_b=0;u_c=0;
    elseif Sa==1 && Sb==0 && Sc==0
        u_alpha=(2/3)*Udc;
        u_b=(-1/3)*Udc;
        u_c=(-1/3)*Udc;
    elseif Sa==1 && Sb==1 && Sc==0
        u_alpha=(1/3)*Udc;
        u_b=(1/3)*Udc;
        u_c=(-2/3)*Udc;
    elseif Sa==0 && Sb==1 && Sc==0
        u_alpha=(-1/3)*Udc;
        u_b=(2/3)*Udc;
        u_c=(-1/3)*Udc;
    elseif Sa==0 && Sb==1 && Sc==1
        u_alpha=(-2/3)*Udc;
        u_b=(1/3)*Udc;
        u_c=(1/3)*Udc;
    elseif Sa==0 && Sb==0 && Sc==1
        u_alpha=(-1/3)*Udc;
        u_b=(-1/3)*Udc;
        u_c=(2/3)*Udc;
    else 
      
        u_alpha=(1/3)*Udc;
        u_b=(-2/3)*Udc;
        u_c=(1/3)*Udc;
    end;

    u_beta=(u_alpha+2*u_b)/sqrt(3);
end;

== matlab function Luenberger/MRAS/CB Estimator/Func ==
  data: Lm input; Lr input; Ls input; Rr input; Rs_e input; K1 output; K2 output; K3 output; Ti output
function [K1,K2,K3,Ti] = fcn(Lm, Lr, Ls, Rr, Rs_e)

Tr=Lr/Rr;

K1=(Lr/Lm)/((Lr*Rs_e/Lm)+(Lm/Tr));
K2=Lm/((Tr*Lr*Rs_e)+(Lm^2));
K3=1/((Lr*Rs_e/Lm)+(Lm/Tr));
Ti=((Ls*Lr)-(Lm^2))/(Lm*((Lr*Rs_e/Lm)+(Lm/Tr)));

== matlab function Luenberger/BO QS LUENBERGER/Luenberger Algorithm/G*I ==
  data: K1 input; GI1 output; K2 input; K3 input; K4 input; GI2 output; GI3 output; GI4 output; eis_alpha input; eis_beta input
function [GI1, GI2, GI3, GI4] = fcn(K1, K2, K3, K4, eis_alpha, eis_beta)

GI1=K1*eis_alpha-K2*eis_beta;
GI2=K2*eis_alpha+K1*eis_beta;
GI3=K3*eis_alpha-K4*eis_beta;
GI4=K4*eis_alpha+K3*eis_beta;

== matlab function Luenberger/BO QS LUENBERGER/Luenberger Algorithm/Gain Matrix ==
  data: Lm input; Lr input; Ls input; Rr input; Rs input; X1 input; AX1 output; X2 input; X3 input; X4 input; w_est input; AX2 output; AX3 output; AX4 output; K1 output; K2 output; K3 output; K4 output
function [AX1, AX2, AX3, AX4, K1, K2, K3, K4] = fcn(Lm, Lr, Ls, Rr, Rs, X1, X2, X3, X4, w_est)

sigma=1-(Lm^2)/(Ls*Lr);

A11=-(Lm^2*Rr+Lr^2*Rs)/(sigma*Ls*Lr^2);% gama
A12=0;
A13=Lm*Rr/(sigma*Ls*Lr^2);
A14=Lm/(sigma*Ls*Lr);
A21=0;
A22=A11;
A23=-A14;
A24=A13;
A31=Lm*Rr/Lr;
A32=0;
A33=-Rr/Lr;
A34=-1;
A41=0;
A42=A31;
A43=-A34;
A44=A33;

AX1=X1*A11+X2*A12+X3*A13+X4*w_est*A14;
AX2=X1*A21+X2*A22+X3*w_est*A23+X4*A24;
AX3=X1*A31+X2*A32+X3*A33+X4*w_est*A34;
AX4=X1*A41+X2*A42+X3*w_est*A43+X4*A44;

%% L matrix
k=1.0001; %1.1

K1=(1-k)*(A11+A33);
K2=(k-1)*w_est;
K3=((k^2-1)*(-A11+A14*A33)+(k-1)*(A11+A33))/A14;
K4=((1-k)/A14)*w_est;

== matlab function Luenberger/BO QS LUENBERGER/Luenberger Adaptation Algorithm/FT/LPF ==
  data: u input; y output
function y = fcn(u)
window_size=10;
beta=0.8;
    
persistent result;

if isempty(result)
    result=zeros(1, window_size);
end

u0=result(1, 1);
tmp=beta*u+(1-beta)*u0;
for i=1:1:(window_size-1)
    result(1, i)=result(1, i+1);
end
result(1, window_size)=2*tmp;

y=tmp;

== matlab function Luenberger/TOC DO DAT/Speed Selection ==
  data: Select input; Speed output; t input
function Speed = fcn(Select, t)

switch Select
    case 1 % 100rpm
        Speed=100;
        
    case 2 % 500rpm
        Speed=500;
        
    otherwise % 1000, 500, 100, 50rpm
        if t<0.75
            Speed=1000;
        elseif t<1.25
            Speed=500;
        else
            Speed=100;
        end
end

== matlab function Luenberger/DTC/DTC ==
  data: Te_fb input; Sa output; Sb output; Sc output; Te_ref input; Flux_ref input; State input; psi_s input; angle input
function [Sa, Sb, Sc] = fcn(Te_fb, Te_ref, Flux_ref, State, psi_s, angle)

HB_Te=0.01;
HB_psi=0.01;

if (Te_ref-Te_fb)>HB_Te,
    H_Te=1;
elseif (Te_ref-Te_fb)<-HB_Te,
    H_Te=-1;
else
    H_Te=0;
end;

H_psi=1;
if (Flux_ref-psi_s)>HB_psi,
    H_psi=1;
end;

if (Flux_ref-psi_s)<-HB_psi,
    H_psi=-1;
end;

Sector=0;
if angle>-30 && angle<=30,
    Sector=1;
elseif angle>30 && angle<=90,
    Sector=2;
elseif angle>90 && angle<=150,
    Sector=3;
elseif angle>150 || angle<=-150,
    Sector=4; 
elseif angle>-150 && angle<=-90,
    Sector=5;
else
    Sector=6;
end;

V=[1 0 0; 1 1 0; 0 1 0; 0 1 1; 0 0 1; 1 0 1; 1 1 1];
if State==0,
    [Sa]=0;
    [Sb]=0;
    [Sc]=0;
else
    if H_psi==1,
        if H_Te==1,
            if Sector<=5,
                [Sa]=V(Sector+1,1);
                [Sb]=V(Sector+1,2);
                [Sc]=V(Sector+1,3);
            else
                [Sa]=V(1,1);
                [Sb]=V(1,2);
                [Sc]=V(1,3);
            end;
        elseif H_Te==-1,
            if Sector>=2 && Sector<=6,
                [Sa]=V(Sector-1,1);
                [Sb]=V(Sector-1,2);
                [Sc]=V(Sector-1,3);
            else
                [Sa]=V(6,1);
                [Sb]=V(6,2);
                [Sc]=V(6,3);
            end;
        else
            [Sa]=V(7,1);
            [Sb]=V(7,2);
            [Sc]=V(7,3);
        end;
    else
        if H_Te==1,
            if Sector<=4,
                [Sa]=V(Sector+2,1);
                [Sb]=V(Sector+2,2);
                [Sc]=V(Sector+2,3);
            else
                [Sa]=V(Sector-4,1);
                [Sb]=V(Sector-4,2);
                [Sc]=V(Sector-4,3);
            end;
        elseif H_Te==-1,
            if Sector>=3 && Sector<=6,
                [Sa]=V(Sector-2,1);
                [Sb]=V(Sector-2,2);
                [Sc]=V(Sector-2,3);
            else
                [Sa]=V(Sector+4,1);
                [Sb]=V(Sector+4,2);
                [Sc]=V(Sector+4,3);
            end;
        else
            [Sa]=V(7,1);
            [Sb]=V(7,2);
            [Sc]=V(7,3);
        end;
    end;
end;

== matlab function Luenberger/BO QS LUENBERGER LPF/Luenberger Adaptation Algorithm/FT/LPF ==
  data: u input; y output
function y = fcn(u)
window_size=10;
beta=0.8;
    
persistent result;

if isempty(result)
    result=zeros(1, window_size);
end

u0=result(1, 1);
tmp=beta*u+(1-beta)*u0;
for i=1:1:(window_size-1)
    result(1, i)=result(1, i+1);
end
result(1, window_size)=2*tmp;

y=tmp;

== matlab function Luenberger/BO QS LUENBERGER LPF/Luenberger Algorithm/G*I ==
  data: K1 input; GI1 output; K2 input; K3 input; K4 input; GI2 output; GI3 output; GI4 output; eis_alpha input; eis_beta input
function [GI1, GI2, GI3, GI4] = fcn(K1, K2, K3, K4, eis_alpha, eis_beta)

GI1=K1*eis_alpha-K2*eis_beta;
GI2=K2*eis_alpha+K1*eis_beta;
GI3=K3*eis_alpha-K4*eis_beta;
GI4=K4*eis_alpha+K3*eis_beta;

== matlab function Luenberger/BO QS LUENBERGER LPF/Luenberger Algorithm/Gain Matrix ==
  data: Lm input; Lr input; Ls input; Rr input; Rs input; X1 input; AX1 output; X2 input; X3 input; X4 input; w_est input; AX2 output; AX3 output; AX4 output; K1 output; K2 output; K3 output; K4 output
function [AX1, AX2, AX3, AX4, K1, K2, K3, K4] = fcn(Lm, Lr, Ls, Rr, Rs, X1, X2, X3, X4, w_est)

sigma=1-(Lm^2)/(Ls*Lr);

A11=-(Lm^2*Rr+Lr^2*Rs)/(sigma*Ls*Lr^2);% gama
A12=0;
A13=Lm*Rr/(sigma*Ls*Lr^2);
A14=Lm/(sigma*Ls*Lr);
A21=0;
A22=A11;
A23=-A14;
A24=A13;
A31=Lm*Rr/Lr;
A32=0;
A33=-Rr/Lr;
A34=-1;
A41=0;
A42=A31;
A43=-A34;
A44=A33;

AX1=X1*A11+X2*A12+X3*A13+X4*w_est*A14;
AX2=X1*A21+X2*A22+X3*w_est*A23+X4*A24;
AX3=X1*A31+X2*A32+X3*A33+X4*w_est*A34;
AX4=X1*A41+X2*A42+X3*w_est*A43+X4*A44;

%% L matrix
k=1.0001; %1.1

K1=(1-k)*(A11+A33);
K2=(k-1)*w_est;
K3=((k^2-1)*(-A11+A14*A33)+(k-1)*(A11+A33))/A14;
K4=((1-k)/A14)*w_est;
